simulink model "SunSensorModel"  (R2018b)
settings: Solver=VariableStepAuto  StartTime=0.0  StopTime=10.0  RelTol=1e-3
undefined symbols (not defined in the file): serial
libraries: instrumentlib x2
settings Model: Creator=Jonathan  LastModifiedBy=Jonathan

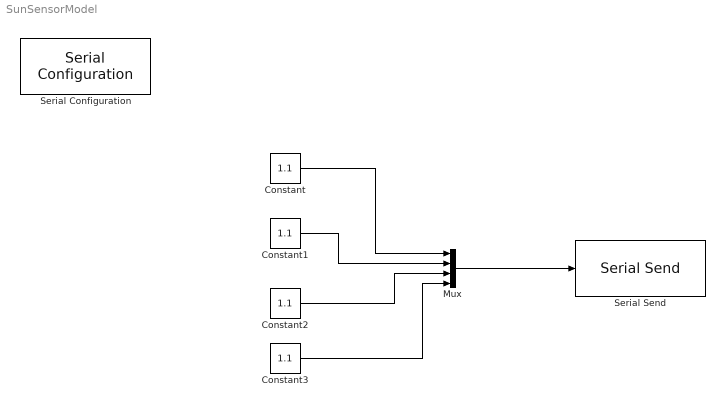
== system SunSensorModel ==
  Constant{,1..3} (4 alike) : Constant  Value=1.1
  Mux : Mux
  Serial Configuration : instrumentlib/Serial Configuration  Priority=-200000  ComPortMenu=COM1  ComPort=COM1  ObjConstructor=serial('COM1');  BaudRate=9600  DataBits=8  Parity=none  StopBits=1  FlowControl=none  Timeout=10  ByteOrder=LittleEndian
  Serial Send : instrumentlib/Serial Send  ComPortMenu=COM1  ComPort=COM1  ObjConstructor=serial('COM1');  Terminator=<none>  EnableBlockingMode=on
  wires:
  Constant/1 -> Mux/1
  Constant1/1 -> Mux/2
  Constant2/1 -> Mux/3
  Constant3/1 -> Mux/4
  Mux/1 -> Serial Send/1
